simulink library "INT_ExtDem_SetPoint"  (R2016b)
settings: Solver=VariableStepAuto  StartTime=0.0  StopTime=10.0  RelTol=1e-3
settings Model: Creator=xuxingpei  LastModifiedBy=xuxingpei

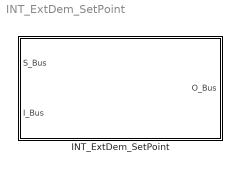
== system INT_ExtDem_SetPoint ==
  INT_ExtDem_SetPoint : Subsystem

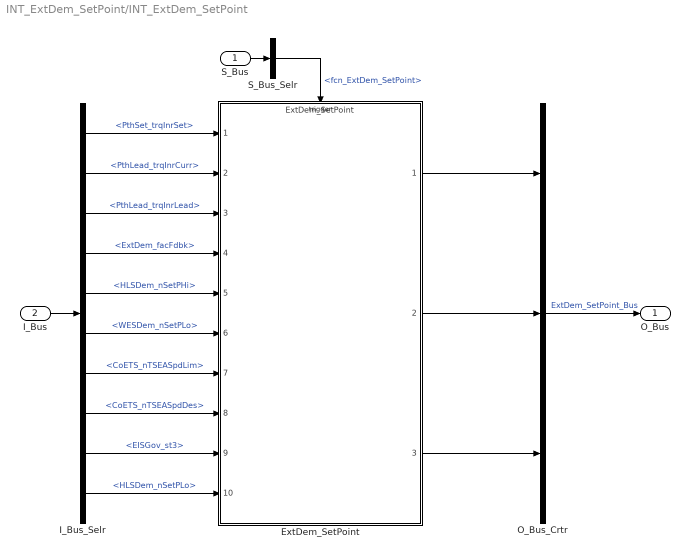
== system INT_ExtDem_SetPoint/INT_ExtDem_SetPoint ==
  S_Bus : Inport
  I_Bus : Inport  Port=2
  ExtDem_SetPoint : ModelReference  ModelNameDialog=ExtDem_SetPoint  SimulationMode=Normal  ModelReferenceVersion=1.44  TriggerPortName=function  TriggerPortTriggerType=function-call  TriggerPortStatesWhenEnabling=held
  I_Bus_Selr : BusSelector  OutputSignals=PthSet_trqInrSet,PthLead_trqInrCurr,PthLead_trqInrLead,ExtDem_facFdbk,HLSDem_nSetPHi,WESDem_nSetPLo,CoETS_nTSEASpdLim,CoETS_nTSEASpdDes,EISGov_st3,HLSDem_nSetPLo
  O_Bus_Crtr : BusCreator  Inputs=3
  S_Bus_Selr : BusSelector  OutputSignals=fcn_ExtDem_SetPoint
  O_Bus : Outport
  wires:
  S_Bus_Selr/1 -> ExtDem_SetPoint/Trigger  "<fcn_ExtDem_SetPoint>"
  S_Bus/1 -> S_Bus_Selr/1
  I_Bus/1 -> I_Bus_Selr/1
  I_Bus_Selr/1 -> ExtDem_SetPoint/1  "<PthSet_trqInrSet>"
  I_Bus_Selr/2 -> ExtDem_SetPoint/2  "<PthLead_trqInrCurr>"
  I_Bus_Selr/3 -> ExtDem_SetPoint/3  "<PthLead_trqInrLead>"
  I_Bus_Selr/4 -> ExtDem_SetPoint/4  "<ExtDem_facFdbk>"
  I_Bus_Selr/5 -> ExtDem_SetPoint/5  "<HLSDem_nSetPHi>"
  I_Bus_Selr/6 -> ExtDem_SetPoint/6  "<WESDem_nSetPLo>"
  I_Bus_Selr/7 -> ExtDem_SetPoint/7  "<CoETS_nTSEASpdLim>"
  I_Bus_Selr/8 -> ExtDem_SetPoint/8  "<CoETS_nTSEASpdDes>"
  I_Bus_Selr/9 -> ExtDem_SetPoint/9  "<EISGov_st3>"
  I_Bus_Selr/10 -> ExtDem_SetPoint/10  "<HLSDem_nSetPLo>"
  O_Bus_Crtr/1 -> O_Bus/1  "ExtDem_SetPoint_Bus"
  ExtDem_SetPoint/1 -> O_Bus_Crtr/1
  ExtDem_SetPoint/2 -> O_Bus_Crtr/2
  ExtDem_SetPoint/3 -> O_Bus_Crtr/3
